simulink subsystem "Single_Channel_Minimum_Jerk"  (R2024a)
settings: Solver=VariableStepAuto  StartTime=0.0  StopTime=10.0  RelTol=1e-3
undefined symbols (not defined in the file): MCU_Ts
libraries: simulink x1
settings Model: DataDictionary=neck_mk3.sldd  EnableAccessToBaseWorkspace=off  Creator=upattacini  LastModifiedBy=upattacini

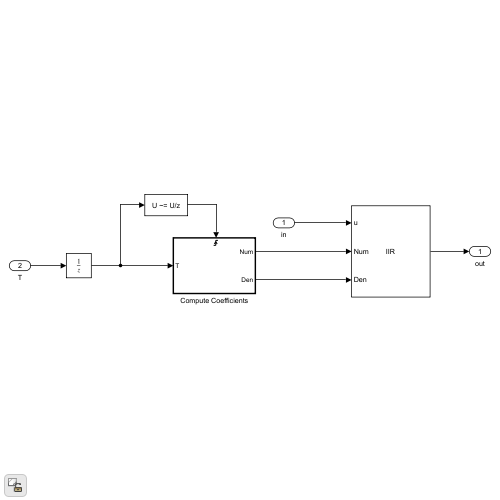
[thumbnail: Simulink's stored preview of the top-level diagram]
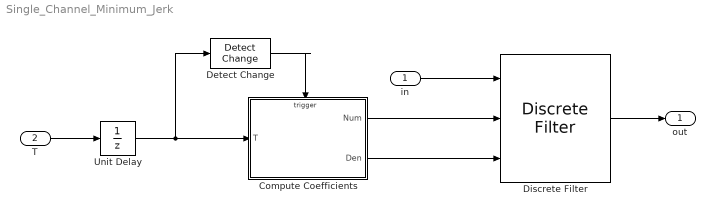
== system Single_Channel_Minimum_Jerk ==
  in : Inport
  T : Inport  Port=2
  Compute Coefficients : Subsystem
  Detect Change : simulink/Logic and Bit Operations/Detect Change  vinit=0  OutDataTypeStr=uint8
  Discrete Filter : DiscreteFilter  NumeratorSource=Input port  DenominatorSource=Input port  a0EqualsOne=on
      settings: InputPortMap=u0,p1,p3
  Unit Delay : UnitDelay  SampleTime=MCU_Ts  HasFrameUpgradeWarning=on
  out : Outport
  wires:
  T/1 -> Unit Delay/1
  Detect Change/1 -> Compute Coefficients/Trigger
  Unit Delay/1 -> Compute Coefficients/1(T), Detect Change/1
  Compute Coefficients/1(Num) -> Discrete Filter/2
  Compute Coefficients/2(Den) -> Discrete Filter/3
  in/1 -> Discrete Filter/1
  Discrete Filter/1 -> out/1

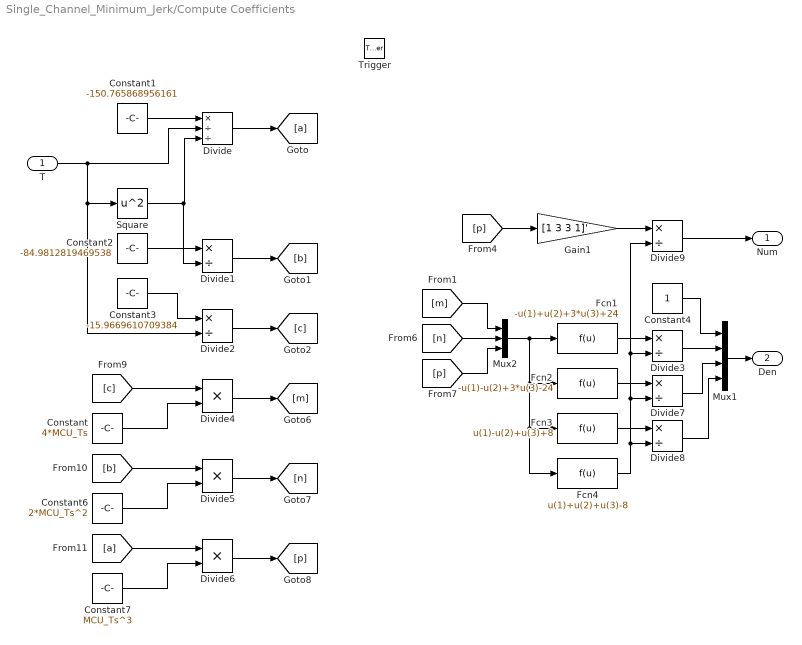
== system Single_Channel_Minimum_Jerk/Compute Coefficients ==
  T : Inport
  Trigger : TriggerPort  VariantControl=(inherit)  PortDimensions=1
  Constant : Constant  Value=4*MCU_Ts
  Constant1 : Constant  Value=-150.765868956161
  Constant2 : Constant  Value=-84.9812819469538
  Constant3 : Constant  Value=-15.9669610709384
  Constant4 : Constant
  Constant6 : Constant  Value=2*MCU_Ts^2
  Constant7 : Constant  Value=MCU_Ts^3
  Divide : Product  Inputs=*//
  Divide{1..3,7..9} (6 alike) : Product  Inputs=*/
  Divide4 : Product  Inputs=**
  Divide5 : Product  Inputs=**
  Divide6 : Product  Inputs=**
  Fcn1 : Fcn  Expr=-u(1)+u(2)+3*u(3)+24
  Fcn2 : Fcn  Expr=-u(1)-u(2)+3*u(3)-24
  Fcn3 : Fcn  Expr=u(1)-u(2)+u(3)+8
  Fcn4 : Fcn  Expr=u(1)+u(2)+u(3)-8
  Gain1 : Gain  Gain=[1 3 3 1]'
  Mux1 : Mux
  Mux2 : Mux  Inputs=3
  Square : Math  Operator=square
  Num : Outport  InitialOutput=[0 0 0 0]
  Den : Outport  Port=2  InitialOutput=[1 0 0 0]'
  wires:
  Divide9/1 -> Num/1
  Gain1/1 -> Divide9/1
  Fcn4/1 -> Divide3/2, Divide9/2, Divide7/2, Divide8/2
  Fcn3/1 -> Divide8/1
  Fcn2/1 -> Divide7/1
  Divide8/1 -> Mux1/4
  Divide7/1 -> Mux1/3
  Divide3/1 -> Mux1/2
  Fcn1/1 -> Divide3/1
  Mux2/1 -> Fcn1/1, Fcn2/1, Fcn3/1, Fcn4/1
  [p] -> Mux2/3
  [n] -> Mux2/2
  [m] -> Mux2/1
  Constant7/1 -> Divide6/2
  [a] -> Divide6/1
  Divide6/1 -> [p]
  Divide5/1 -> [n]
  [b] -> Divide5/1
  Constant6/1 -> Divide5/2
  Constant/1 -> Divide4/2
  [c] -> Divide4/1
  Divide4/1 -> [m]
  Mux1/1 -> Den/1
  Constant4/1 -> Mux1/1
  Divide/1 -> [a]
  Square/1 -> Divide/3, Divide1/2
  Constant3/1 -> Divide2/1
  Constant2/1 -> Divide1/1
  [p] -> Gain1/1
  Divide2/1 -> [c]
  T/1 -> Divide/2, Square/1, Divide2/2
  Divide1/1 -> [b]
  Constant1/1 -> Divide/1
